simulink subsystem "Mk2MotorDrivers_Ideal"  (R2025a)
settings: Solver=VariableStepAuto  StartTime=0.0  StopTime=10.0  RelTol=1e-3
undefined symbols (not defined in the file): Phase1_Pos, Phase2_Pos, Phase3_Pos, Phase_Neg
libraries: fl_lib x1
settings Model: DataDictionary=neck_mk3.sldd  EnableAccessToBaseWorkspace=off  Creator=upattacini  LastModifiedBy=upattacini
settings RTWCC: GPUComputeCapability=3.5

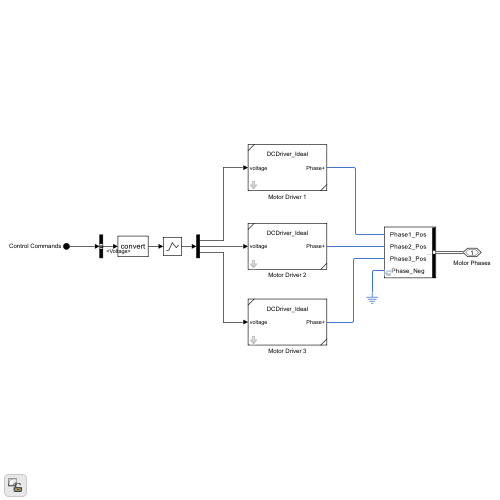
[thumbnail: Simulink's stored preview of the top-level diagram]
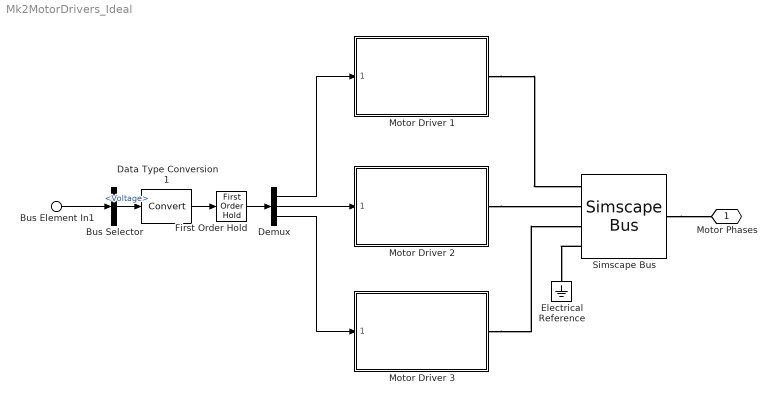
== system Mk2MotorDrivers_Ideal ==
  Bus Element In1 : Inport  PortName=Control Commands
  Bus Selector : BusSelector  OutputSignals=Voltage
  Data Type Conversion1 : DataTypeConversion  SaturateOnIntegerOverflow=off  RndMeth=Floor
  Demux : Demux  Outputs=3
  Electrical Reference : fl_lib/Electrical/Electrical Elements/Electrical Reference
  First Order Hold : FirstOrderHold  ErrorTolerance=inf
  Motor Driver 1 : Subsystem  ReferencedSubsystem=DCDriver_Ideal  Supply_Vcc=12
      settings: PermitHierarchicalResolution=None
  Motor Driver 2 : Subsystem  ReferencedSubsystem=DCDriver_Ideal  Supply_Vcc=12
      settings: PermitHierarchicalResolution=None
  Motor Driver 3 : Subsystem  ReferencedSubsystem=DCDriver_Ideal  Supply_Vcc=12
      settings: PermitHierarchicalResolution=None
  Simscape Bus : SimscapeBus  HierarchyStrings=Phase1_Pos;Phase2_Pos;Phase3_Pos;Phase_Neg  ConnectionType=Bus: Physical_MotorPhases
  Motor Phases : PMIOPort  Side=Right  ConnectionType=Bus: Physical_MotorPhases
  wires:
  Bus Element In1/1 -> Bus Selector/1
  Bus Selector/1 -> Data Type Conversion1/1  "<Voltage>"
  Demux/1 -> Motor Driver 1/1
  Demux/2 -> Motor Driver 2/1
  Demux/3 -> Motor Driver 3/1
  First Order Hold/1 -> Demux/1
  Data Type Conversion1/1 -> First Order Hold/1
  connections:
  Simscape Bus/RConn1 -- Motor Phases/RConn1
  Motor Driver 1/RConn1 -- Simscape Bus/LConn1
  Motor Driver 2/RConn1 -- Simscape Bus/LConn2
  Motor Driver 3/RConn1 -- Simscape Bus/LConn3
  Simscape Bus/LConn4 -- Electrical Reference/LConn1
